simulink model "teste_ma"  (R2013a)
settings: Solver=ode45  StartTime=0.0  StopTime=Tsim  RelTol=1e-3
values from neighbouring files (symbols this model uses):
  dist = 5    [load_variables.m]    (also in matlab.mat; matlab2.mat; matlab_workspace.mat)
  ref = 10    [load_variables.m]    (also in matlab.mat; matlab2.mat; matlab_workspace.mat)
  Tref = 800    [load_variables.m]    (also in matlab.mat = 600; matlab2.mat = 600; matlab_workspace.mat = 700)
  Trefdown = Tref+Tstepdown    (= 2420)    [load_variables.m]    (also in matlab.mat = 2400; matlab2.mat = 2400; matlab_workspace.mat = 2500)
  Ts = 5    [load_variables.m]    (also in matlab.mat; matlab2.mat; matlab_workspace.mat)
  Tsim = Tref+Trefdown    (= 3220)    [load_variables.m]    (also in matlab.mat = 800; matlab2.mat = 800; matlab_workspace.mat = 3200)
  Tstep = 2*Tref    (= 1600)    [load_variables.m]    (also in matlab_workspace.mat)
  Tstepdown = Tstep+Thold    (= 1620)    [load_variables.m]    (also in matlab_workspace.mat = 2000)
libraries: opclib x3, commchan3 x1, cstblocks x1
settings Model: Creator=didaticontrol  LastModifiedBy=didaticontrol

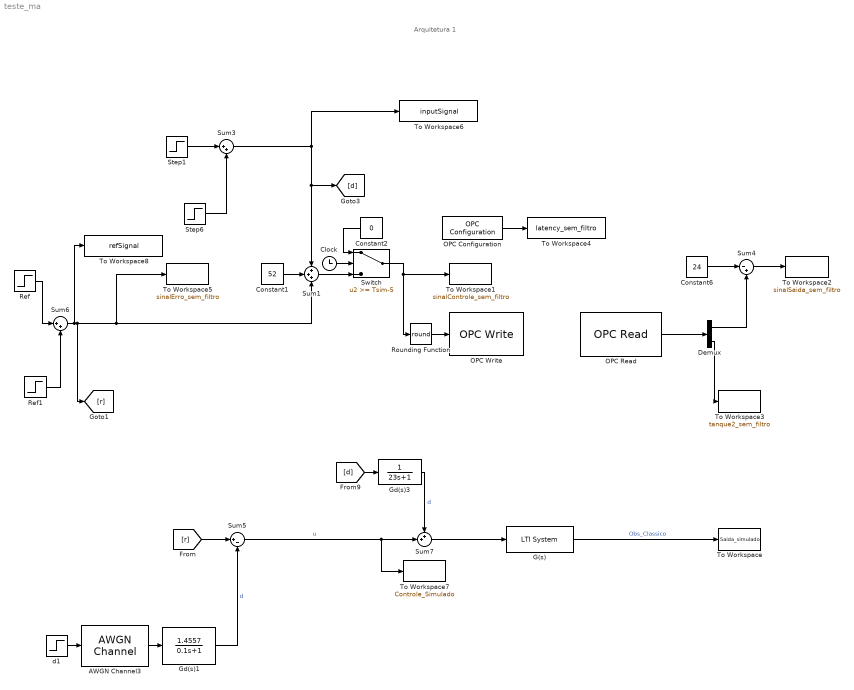
== system teste_ma ==
  note: Arquitetura 1
  AWGN Channel3 : commchan3/AWGN Channel  InputProcessing=Columns as channels (frame based)  seed=67  noiseMode=Variance from mask  EbNodB=10  EsNodB=10  SNRdB=10  bitsPerSym=1  Ps=1  Tsym=1  variance=var_ruido
  Clock : Clock
  Constant1 : Constant  Value=52
  Constant2 : Constant  Value=0
  Constant6 : Constant  Value=24
  Demux : Demux  Outputs=2
  G(s) : cstblocks/LTI System  sys=Gs  IC=[]
  Gd(s)1 : TransferFcn  Numerator=1.4557  Denominator=[0.1 1]
  Gd(s)3 : TransferFcn  Numerator=1  Denominator=[23 1]
  OPC Configuration : opclib/OPC Configuration  opcServers=143.106.123.105/BR.OPC.Server_AR/10  errMissingItems=Error  errReadWrite=Warn  errShutdown=Error  errRTViolation=Warn  rtEnable=on  speedup=1  showLatency=on  beingUsed=on
  OPC Read : opclib/OPC Read  serverHost=143.106.123.105  serverID=BR.OPC.Server_AR  itemIDs=PTQ4_corrigido, PTQ2_corrigido  readMode=Synchronous (cache)  dataType=double  updateRate=5  showQual=off  showTS=off  tsMode=Seconds since start
  OPC Write : opclib/OPC Write  serverHost=143.106.123.105  serverID=BR.OPC.Server_AR  itemIDs=Bomba2  writeMode=Synchronous  updateRate=-1
  Ref : Step  Time=Tref  After=ref  SampleTime=0
  Ref1 : Step  Time=Trefdown  After=-ref  SampleTime=0
  Rounding Function : Rounding  Operator=round
  Step1 : Step  Time=Tstep  After=dist  SampleTime=0
  Step6 : Step  Time=Tstepdown  After=-dist  SampleTime=0
  Sum1 : Sum  Inputs=+++
  Sum3 : Sum  Inputs=|++
  Sum4 : Sum  Inputs=|-+
  Sum5 : Sum  Inputs=|+-
  Sum6 : Sum  Inputs=|++
  Sum7 : Sum  Inputs=++|
  Switch : Switch  Threshold=Tsim-5
  To Workspace : ToWorkspace  VariableName=Saida_simulado  SampleTime=-1  SaveFormat=Timeseries
  To Workspace1 : ToWorkspace  VariableName=sinalControle_sem_filtro  SampleTime=Ts  SaveFormat=Timeseries
  To Workspace2 : ToWorkspace  VariableName=sinalSaida_sem_filtro  SampleTime=Ts  SaveFormat=Timeseries
  To Workspace3 : ToWorkspace  VariableName=tanque2_sem_filtro  SampleTime=Ts  SaveFormat=Timeseries
  To Workspace4 : ToWorkspace  VariableName=latency_sem_filtro  SampleTime=Ts  SaveFormat=Timeseries
  To Workspace5 : ToWorkspace  VariableName=sinalErro_sem_filtro  SampleTime=Ts  SaveFormat=Timeseries
  To Workspace6 : ToWorkspace  VariableName=inputSignal  SampleTime=Ts  SaveFormat=Timeseries
  To Workspace7 : ToWorkspace  VariableName=Controle_Simulado  SampleTime=-1  SaveFormat=Timeseries
  To Workspace8 : ToWorkspace  VariableName=refSignal  SampleTime=Ts  SaveFormat=Timeseries
  d1 : Step  Time=0  After=0  SampleTime=Ts
  wires:
  Constant6/1 -> Sum4/1
  Sum4/1 -> To Workspace2/1
  OPC Read/1 -> Demux/1
  Demux/1 -> Sum4/2
  Demux/2 -> To Workspace3/1
  OPC Configuration/1 -> To Workspace4/1
  Sum3/1 -> [d], Sum1/1, To Workspace6/1
  Step6/1 -> Sum3/2
  Step1/1 -> Sum3/1
  Sum6/1 -> To Workspace8/1, Sum1/3, To Workspace5/1, [r]
  Constant1/1 -> Sum1/2
  Rounding Function/1 -> OPC Write/1
  [r] -> Sum5/1
  Sum7/1 -> G(s)/1
  G(s)/1 -> To Workspace/1  "Obs_Classico"
  [d] -> Gd(s)3/1
  Gd(s)3/1 -> Sum7/1  "d"
  Sum5/1 -> Sum7/2, To Workspace7/1  "u"
  Ref/1 -> Sum6/1
  Ref1/1 -> Sum6/2
  Switch/1 -> Rounding Function/1, To Workspace1/1
  Sum1/1 -> Switch/3
  Clock/1 -> Switch/2
  Constant2/1 -> Switch/1
  d1/1 -> AWGN Channel3/1
  AWGN Channel3/1 -> Gd(s)1/1
  Gd(s)1/1 -> Sum5/2  "d"
